simulink model "Gestione_Agricola"  (R2023b)
settings: Solver=VariableStepAuto  StartTime=0.0  StopTime=120.0  RelTol=1e-3
undefined symbols (not defined in the file or in its folder): ZigBee
libraries: truetime x13, fuzblock x1
settings Model: Creator=giovanni02  LastModifiedBy=francescopaoloseverino

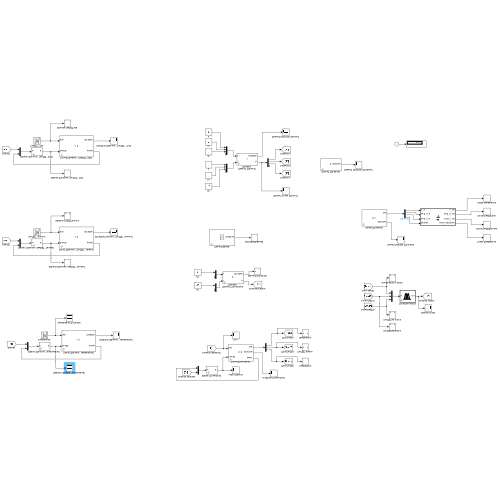
[thumbnail: Simulink's stored preview of the top-level diagram]
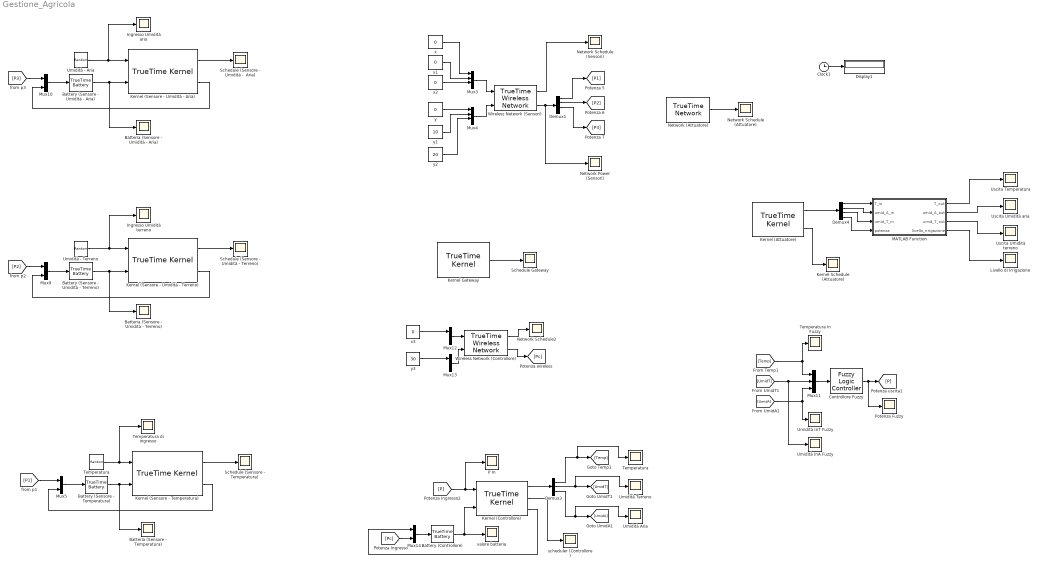
== system Gestione_Agricola ==
  Batteria (Sensore - Temperatura) : Scope
  Batteria (Sensore - Umidità - Aria) : Scope
  Batteria (Sensore - Umidità - Terreno) : Scope
  Battery (Controllore) : truetime/TrueTime Battery  energy=10000
  "Battery (Sensore - Temperatura) " : truetime/TrueTime Battery  energy=10000
  Battery (Sensore - Umidità - Aria) : truetime/TrueTime Battery  energy=10000
  "Battery (Sensore - Umidità - Terreno) " : truetime/TrueTime Battery  energy=10000
  Clock1 : Clock
  Controllore Fuzzy : fuzblock/Fuzzy Logic  Controller  FIS='ControlloreFuzzy.fis'  OutputSampleNumber=101  DataType=double  FuzzifiedInputs=off  RuleFiringStrengths=off  RuleOutputs=off  AggregatedOutputs=off  SimulateUsing=Interpreted execution  OutOfRangeInputValueMessage=warning  NoRuleFiredMessage=warning  EmptyOutputFuzzySetMessage=warning
  Demux1 : Demux
  Demux3 : Demux  Outputs=3
  Demux4 : Demux
  Display1 : Display
  Ingresso Umidità aria : Scope
  Ingresso Umidità terreno : Scope
  Kernel (Attuatore) : truetime/TrueTime Kernel  sfun=Attuatore_init  args=[]  ninputsoutputs=[0 4]  ntriggers=0  trigtype=falling  nwnodenbr=[3 1]  clockoffsetdrift=[0 0]  schedoutput=on  battery=off  poweroutput=off  label=3: 1
  Kernel (Controllore) : truetime/TrueTime Kernel  sfun=Controllore_init  args=[]  ninputsoutputs=[1 3]  ntriggers=0  trigtype=falling  nwnodenbr=[2 2]  clockoffsetdrift=[0 0]  schedoutput=on  battery=on  poweroutput=on  label=2: 2
  Kernel (Sensore - Temperatura) : truetime/TrueTime Kernel  sfun=Sensore_temperatura_init  args=[]  ninputsoutputs=[1 0]  ntriggers=0  trigtype=falling  nwnodenbr=[1 1]  clockoffsetdrift=[0 0]  schedoutput=on  battery=on  poweroutput=on  label=1: 1
  Kernel (Sensore - Umidità - Aria) : truetime/TrueTime Kernel  sfun=Sensore_umidita_aria_init  args=[]  ninputsoutputs=[1 0]  ntriggers=0  trigtype=falling  nwnodenbr=[1 3]  clockoffsetdrift=[0 0]  schedoutput=on  battery=on  poweroutput=on  label=1: 3
  Kernel (Sensore - Umidità - Terreno) : truetime/TrueTime Kernel  sfun=Sensore_umidita_terreno_init  args=[]  ninputsoutputs=[1 0]  ntriggers=0  trigtype=falling  nwnodenbr=[1 2]  clockoffsetdrift=[0 0]  schedoutput=on  battery=on  poweroutput=on  label=1: 2
  Kernel Gateway : truetime/TrueTime Kernel  sfun=Gateway_init  args=[]  ninputsoutputs=[0 0]  ntriggers=0  trigtype=falling  nwnodenbr=[1 4; 2 4; 3 4]  clockoffsetdrift=[0 0]  schedoutput=on  battery=off  poweroutput=off  label=1: 4\n2: 4\n3: 4
  Kernel Schedule (Attuatore) : Scope
  Livello di Irrigazione : Scope
  MATLAB Function : MATLAB Function  TreatAsAtomicUnit=on
  Mux{5,9..10,12..14} (6 alike) : Mux  Inputs=2
  Mux11 : Mux  Inputs=3
  Mux3 : Mux
  Mux4 : Mux
  Network (Attuatore) : truetime/TrueTime Network  nwtype=CSMA/CD (Ethernet)  nwnbr=3  nnodes=4  rate=10000000  minsize=512  lossprob=0  seed=0  bandwidths=[0.5 0.5]  slotsize=512  schedule=[1 1 2]  memsize=80000  buftype=Common buffer  overflow=Retransmit  dynSchedule=0  miniSlotSize=0  NIT=0  QSortMode=FIFO  sync=0  irtSchedule=0  nrtLength=0  nodeGraph=0  scheduleoutput=on
  Network Power (Sensori) : Scope
  Network Schedule (Attuatore) : Scope
  Network Schedule (Sensori) : Scope
  Network Schedule2 : Scope
  P In : Scope
  Potenza Fuzzy : Scope
  Schedule (Sensore - Temperatura) : Scope
  Schedule (Sensore - Umidità -  Aria) : Scope
  Schedule (Sensore - Umidità - Terreno) : Scope
  Schedule Gateway : Scope
  Temperatura : UniformRandomNumber  Minimum=15  Maximum=40  SampleTime=1
  "Temperatura " : Scope
  Temperatura In Fuzzy : Scope
  Temperatura di ingresso : Scope
  Umidità - Aria : UniformRandomNumber  Minimum=30  Maximum=90  SampleTime=1
  Umidità - Terreno : UniformRandomNumber  Minimum=30  Maximum=90  SampleTime=1
  Umidità Aria : Scope
  Umidità InA Fuzzy : Scope
  Umidità InT Fuzzy : Scope
  Umidità Terreno : Scope
  Uscita Temperatura : Scope
  Uscita Umidità aria : Scope
  Uscita Umidità terreno : Scope
  Wireless Network (Controllore) : truetime/TrueTime Wireless  Network  nwtype=802.15.4 (ZigBee)  nwnbr=2  nnodes=4  rate=800000  minsize=272  transpower=20  threshold=-48  use_pathloss_function=default  pathloss=3.5  acktimeout=0.00004  retrylimit=5  error_threshold=0.03  lossprob=0  seed=0  scheduleoutput=on  poweroutput=on
  Wireless Network (Sensori) : truetime/TrueTime Wireless  Network  nwtype=802.15.4 (ZigBee)  nwnbr=1  nnodes=4  rate=800000  minsize=272  transpower=20  threshold=-48  use_pathloss_function=default  pathloss=3.5  acktimeout=0.00004  retrylimit=5  error_threshold=0.03  lossprob=0  seed=0  scheduleoutput=on  poweroutput=on
  scheduler (Controllore) : Scope
  valore batteria : Scope
  x{,1..3} (4 alike) : Constant  Value=0
  y : Constant  Value=0
  y1 : Constant  Value=10
  y2 : Constant  Value=20
  y3 : Constant  Value=30
  wires:
  Kernel Gateway/1 -> Schedule Gateway/1
  "Battery (Sensore - Temperatura) "/1 -> Kernel (Sensore - Temperatura)/2, Batteria (Sensore - Temperatura)/1
  Network (Attuatore)/1 -> Network Schedule (Attuatore)/1
  Mux11/1 -> Controllore Fuzzy/1
  Mux3/1 -> Wireless Network (Sensori)/1
  Kernel (Controllore)/1 -> Demux3/1
  Mux12/1 -> Wireless Network (Controllore)/1
  MATLAB Function/1(T_out) -> Uscita Temperatura/1
  Kernel (Sensore - Temperatura)/1 -> Schedule (Sensore - Temperatura)/1
  [UmidT] -> Umidità InA Fuzzy/1, Mux11/2
  Battery (Sensore - Umidità - Aria)/1 -> Kernel (Sensore - Umidità - Aria)/2, Batteria (Sensore - Umidità - Aria)/1
  Temperatura/1 -> Kernel (Sensore - Temperatura)/1, Temperatura di ingresso/1
  Mux9/1 -> "Battery (Sensore - Umidità - Terreno) "/1
  y2/1 -> Mux4/3
  [UmidA] -> Umidità InT Fuzzy/1, Mux11/3
  Wireless Network (Sensori)/2 -> Demux1/1, Network Power (Sensori)/1
  Wireless Network (Sensori)/1 -> Network Schedule (Sensori)/1
  Clock1/1 -> Display1/1
  MATLAB Function/3(umid_T_out) -> Uscita Umidità terreno/1
  Wireless Network (Controllore)/1 -> Network Schedule2/1
  Mux13/1 -> Wireless Network (Controllore)/2
  Demux1/2 -> [P2]
  Kernel (Sensore - Umidità - Aria)/1 -> Schedule (Sensore - Umidità -  Aria)/1
  Wireless Network (Controllore)/2 -> [Pc]
  [Temp] -> Mux11/1, Temperatura In Fuzzy/1
  x3/1 -> Mux12/1
  [P2] -> Mux9/1
  Demux1/3 -> [P3]
  Kernel (Attuatore)/1 -> Demux4/1
  Kernel (Controllore)/3 -> Mux14/1
  [P] -> P In/1, Kernel (Controllore)/1
  x/1 -> Mux3/1
  Demux4/3 -> MATLAB Function/3(umid_T_in)
  "Battery (Sensore - Umidità - Terreno) "/1 -> Kernel (Sensore - Umidità - Terreno)/2, Batteria (Sensore - Umidità - Terreno)/1
  Demux3/1 -> "Temperatura "/1, [Temp]
  [P1] -> Mux5/1
  Mux5/1 -> "Battery (Sensore - Temperatura) "/1
  Kernel (Sensore - Temperatura)/2 -> Mux5/2
  Umidità - Terreno/1 -> Kernel (Sensore - Umidità - Terreno)/1, Ingresso Umidità terreno/1
  Demux4/1 -> MATLAB Function/1(T_in)
  Kernel (Sensore - Umidità - Terreno)/2 -> Mux9/2
  Mux4/1 -> Wireless Network (Sensori)/2
  y1/1 -> Mux4/2
  y3/1 -> Mux13/1
  Kernel (Sensore - Umidità - Terreno)/1 -> Schedule (Sensore - Umidità - Terreno)/1
  Kernel (Attuatore)/2 -> Kernel Schedule (Attuatore)/1
  Umidità - Aria/1 -> Kernel (Sensore - Umidità - Aria)/1, Ingresso Umidità aria/1
  Kernel (Controllore)/2 -> scheduler (Controllore)/1
  Controllore Fuzzy/1 -> Potenza Fuzzy/1, [P]
  Mux14/1 -> Battery (Controllore)/1
  [P3] -> Mux10/1
  Battery (Controllore)/1 -> valore batteria/1, Kernel (Controllore)/2
  y/1 -> Mux4/1
  Demux3/2 -> [UmidT], Umidità Terreno/1
  [Pc] -> Mux14/2
  Mux10/1 -> Battery (Sensore - Umidità - Aria)/1
  x2/1 -> Mux3/3
  Kernel (Sensore - Umidità - Aria)/2 -> Mux10/2
  Demux3/3 -> [UmidA], Umidità Aria/1
  Demux1/1 -> [P1]
  Demux4/4 -> MATLAB Function/4(potenza)
  MATLAB Function/2(umid_A_out) -> Uscita Umidità aria/1
  MATLAB Function/4(livello_irrigazione) -> Livello di Irrigazione/1
  Demux4/2 -> MATLAB Function/2(umid_A_in)
  x1/1 -> Mux3/2

== matlab function Gestione_Agricola/MATLAB Function ==
  data: T_in input; T_out output; umid_A_in input; umid_T_in input; potenza input; umid_A_out output; umid_T_out output; livello_irrigazione output
function [T_out, umid_A_out, umid_T_out, livello_irrigazione] = fcn(T_in, umid_A_in, umid_T_in, potenza)
umid_A_out = umid_A_in;
umid_T_out = umid_T_in;
T_out = T_in;
livello_irrigazione = 0;

if potenza >= 6
    while umid_A_out > 55.5 && umid_T_out > 52.5
        umid_A_out = umid_A_out - potenza * 1.5;
        umid_T_out = umid_T_out - potenza * 1.5;
        %disp('valore umidita terreno uscita:');
        %disp(umid_T_out);
    end

    if T_in >= 25.5
        while T_out > 20
            T_out = T_out - potenza * 1.5;
            %disp('valore temperatura uscita:');
            %disp(T_out);
        end
    end
    

    livello_irrigazione = 0;

elseif potenza >= 4 && potenza < 6
    if T_in >= 25.5
        while T_out > 20
            T_out = T_out - potenza * 1.5;
            %disp('valore temperatura 2 uscita:');
            %disp(T_out);
        end
    end

    if umid_T_in > 38
        umid_T_out = umid_T_out - potenza;
    end

    if umid_A_in > 35
        umid_A_out = umid_A_out - potenza;
    end

    livello_irrigazione = 1;

elseif potenza < 4
    umid_A_out = umid_A_out + potenza;
    umid_T_out = umid_T_out + potenza;

    if T_in <= 15
        T_out = T_out + potenza * 1.5;
    end

    livello_irrigazione = 0;
    disp(livello_irrigazione);
end
